simulink model "throttle_valve_dynamics"  (R2023a)
settings: Solver=ode45  StartTime=0.0  StopTime=10.0  MaxStep=1e-2  RelTol=1e-3
undefined symbols (not defined in the file): cF, cM, cn, cphi, iG, Jges, LA, MFv, MH, phi0, phi30, phimax, phiminV, phip30, RA, TADC, TSample, TSensor, UB
settings Model: Creator=Sascha  LastModifiedBy=Sascha
settings SolverCC: AlgebraicLoopSolver=TrustRegion
settings DebuggingCC: UnconnectedInputMsg=warning  UnconnectedOutputMsg=warning  UnconnectedLineMsg=warning
settings ModelReferenceCC: EnableRefExpFcnMdlSchedulingChecks=on
settings RTWCC: DLArmComputeVersion=19.05

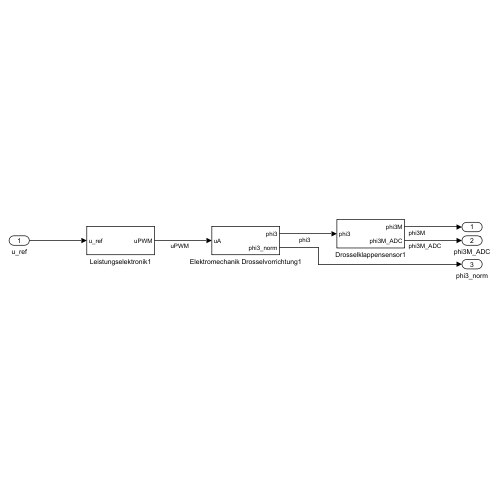
[thumbnail: Simulink's stored preview of the top-level diagram]
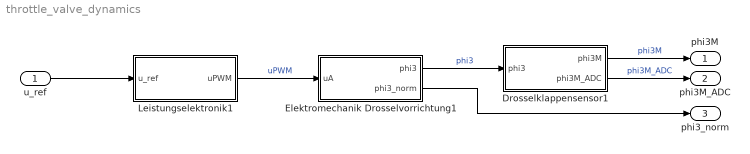
== system throttle_valve_dynamics ==
  u_ref : Inport
  Drosselklappensensor1 : Subsystem
  Elektromechanik Drosselvorrichtung1 : Subsystem
  Leistungselektronik1 : Subsystem
  phi3M : Outport
  phi3M_ADC : Outport  Port=2
  phi3_norm : Outport  Port=3
  wires:
  Elektromechanik Drosselvorrichtung1/2(phi3_norm) -> phi3_norm/1
  u_ref/1 -> Leistungselektronik1/1(u_ref)
  Drosselklappensensor1/2(phi3M_ADC) -> phi3M_ADC/1  "phi3M_ADC"
  Elektromechanik Drosselvorrichtung1/1(phi3) -> Drosselklappensensor1/1(phi3)  "phi3"
  Leistungselektronik1/1(uPWM) -> Elektromechanik Drosselvorrichtung1/1(uA)  "uPWM"
  Drosselklappensensor1/1(phi3M) -> phi3M/1  "phi3M"

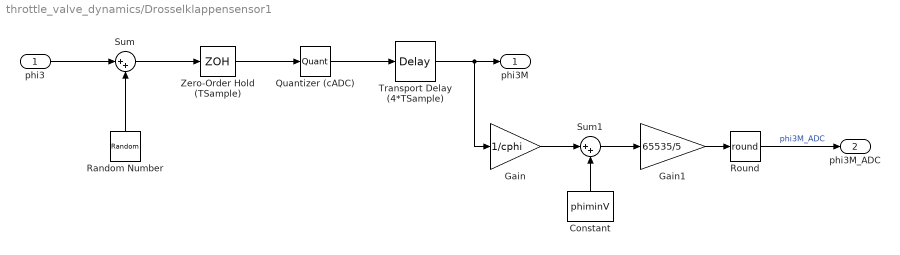
== system throttle_valve_dynamics/Drosselklappensensor1 ==
  phi3 : Inport
  Constant : Constant  Value=phiminV
  Gain : Gain  Gain=1/cphi
  Gain1 : Gain  Gain=65535/5
  Quantizer (cADC) : Quantizer  QuantizationInterval=cADC
  Random Number : RandomNumber  Variance=0.0000015  Seed=5  SampleTime=TADC
  Round : Rounding  Operator=round
  Sum : Sum  Inputs=|++
  Sum1 : Sum  Inputs=|++
  Transport Delay (4*TSample) : TransportDelay  DelayTime=TSensor  InitialOutput=phi0
  Zero-Order Hold (TSample) : ZeroOrderHold  SampleTime=TADC
  phi3M : Outport
  phi3M_ADC : Outport  Port=2
  wires:
  phi3/1 -> Sum/1
  Zero-Order Hold (TSample)/1 -> Quantizer (cADC)/1
  Quantizer (cADC)/1 -> Transport Delay (4*TSample)/1
  Random Number/1 -> Sum/2
  Sum/1 -> Zero-Order Hold (TSample)/1
  Round/1 -> phi3M_ADC/1  "phi3M_ADC"
  Gain/1 -> Sum1/1
  Constant/1 -> Sum1/2
  Sum1/1 -> Gain1/1
  Transport Delay (4*TSample)/1 -> Gain/1, phi3M/1
  Gain1/1 -> Round/1

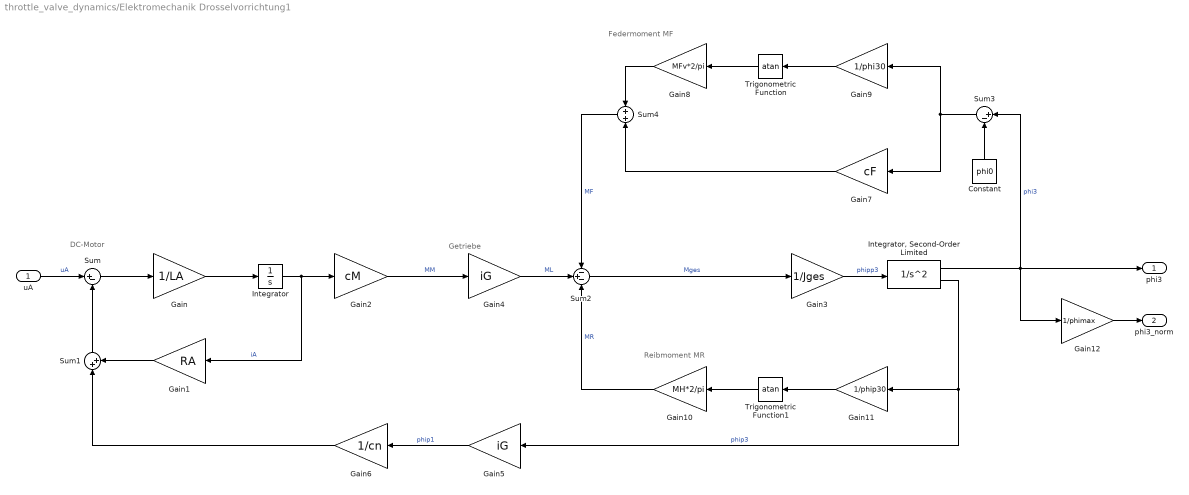
== system throttle_valve_dynamics/Elektromechanik Drosselvorrichtung1 ==
  note: Getriebe
  note: DC-Motor
  note: Reibmoment MR
  note: Federmoment MF
  uA : Inport
  Constant : Constant  Value=phi0
  Gain : Gain  Gain=1/LA
  Gain1 : Gain  Gain=RA
  Gain10 : Gain  Gain=MH*2/pi
  Gain11 : Gain  Gain=1/phip30
  Gain12 : Gain  Gain=1/phimax
  Gain2 : Gain  Gain=cM
  Gain3 : Gain  Gain=1/Jges
  Gain4 : Gain  Gain=iG
  Gain5 : Gain  Gain=iG
  Gain6 : Gain  Gain=1/cn
  Gain7 : Gain  Gain=cF
  Gain8 : Gain  Gain=MFv*2/pi
  Gain9 : Gain  Gain=1/phi30
  Integrator : Integrator
  "Integrator, Second-Order Limited" : SecondOrderIntegrator  ICX=phi0  LimitX=on  UpperLimitX=phimax  LowerLimitX=phimin  StateNameX='phi'  StateNameDXDT='phip'  ReinitDXDTwhenXreachesSaturation=on
  Sum : Sum  Inputs=|+-
  Sum1 : Sum  Inputs=|++
  Sum2 : Sum  Inputs=-+-
  Sum3 : Sum  Inputs=|+-
  Sum4 : Sum  Inputs=+|+
  Trigonometric Function : Trigonometry  Operator=atan
  Trigonometric Function1 : Trigonometry  Operator=atan
  phi3 : Outport
  phi3_norm : Outport  Port=2
  wires:
  uA/1 -> Sum/1  "uA"
  Sum/1 -> Gain/1
  Gain/1 -> Integrator/1
  Integrator/1 -> Gain2/1, Gain1/1  "iA"
  Gain1/1 -> Sum1/2
  Sum1/1 -> Sum/2
  Gain2/1 -> Gain4/1  "MM"
  Gain4/1 -> Sum2/2  "ML"
  Sum2/1 -> Gain3/1  "Mges"
  Gain3/1 -> "Integrator, Second-Order Limited"/1  "phipp3"
  "Integrator, Second-Order Limited"/2 -> Gain11/1, Gain5/1  "phip3"
  "Integrator, Second-Order Limited"/1 -> Gain12/1, Sum3/1, phi3/1  "phi3"
  Gain5/1 -> Gain6/1  "phip1"
  Gain6/1 -> Sum1/1
  Constant/1 -> Sum3/2
  Gain7/1 -> Sum4/2
  Sum3/1 -> Gain9/1, Gain7/1
  Sum4/1 -> Sum2/1  "MF"
  Trigonometric Function/1 -> Gain8/1
  Gain9/1 -> Trigonometric Function/1
  Gain11/1 -> Trigonometric Function1/1
  Trigonometric Function1/1 -> Gain10/1
  Gain8/1 -> Sum4/1
  Gain10/1 -> Sum2/3  "MR"
  Gain12/1 -> phi3_norm/1

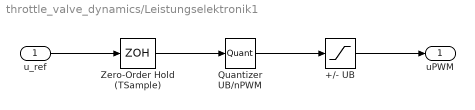
== system throttle_valve_dynamics/Leistungselektronik1 ==
  u_ref : Inport
  +/- UB : Saturate  UpperLimit=UB  LowerLimit=-UB
  Quantizer UB/nPWM : Quantizer  QuantizationInterval=cPWM
  Zero-Order Hold (TSample) : ZeroOrderHold  SampleTime=TSample
  uPWM : Outport
  wires:
  u_ref/1 -> Zero-Order Hold (TSample)/1
  Quantizer UB/nPWM/1 -> +/- UB/1
  +/- UB/1 -> uPWM/1
  Zero-Order Hold (TSample)/1 -> Quantizer UB/nPWM/1
